simulink model "Pcontrol_perturbed"  (R2024b)
settings: Solver=ode4  StartTime=0.0  StopTime=T  FixedStep=Ts  RelTol=1e-3
values from neighbouring files (symbols this model uses):
  C_perturb = eye(5)    [IP_MACRO.m]
  D_perturb = [0 0 0 0 0]'    [IP_MACRO.m]
  K = lqr(A, B, Qr, Rr)    [IP_MACRO.m]
  x0 = [0.1 1 0.2 0 0]'    [IP_MACRO.m]
undefined symbols (not defined in the file or in its folder): A, B
settings Model: Creator=leita  LastModifiedBy=leita
settings DataIOCC: ReturnWorkspaceOutputs=off

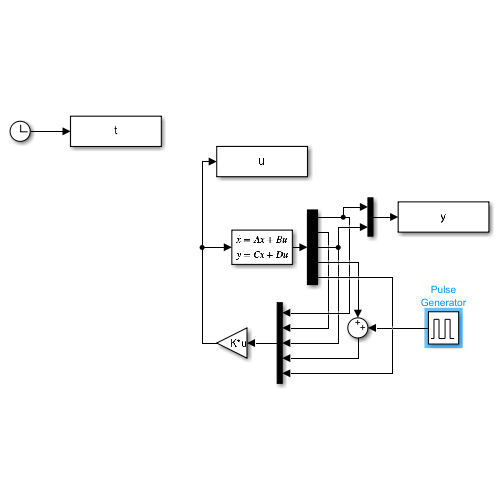
[thumbnail: Simulink's stored preview of the top-level diagram]
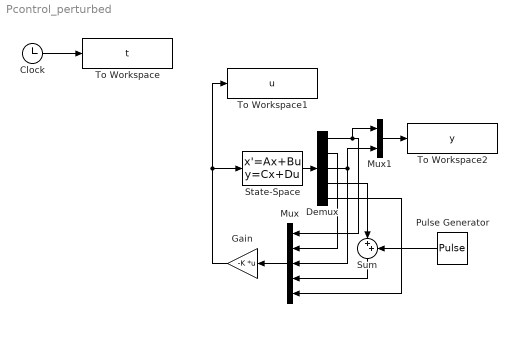
== system Pcontrol_perturbed ==
  Clock : Clock
  Demux : Demux  Outputs=5
  Gain : Gain  Gain=-K  Multiplication=Matrix(K*u)
  Mux : Mux  Inputs=5
  Mux1 : Mux  Inputs=2
  Pulse Generator : DiscretePulseGenerator  PulseType=Time based  Amplitude=5  Period=1  PulseWidth=0.5
  State-Space : StateSpace  A=A  B=B  C=C_perturb  D=D_perturb  InitialCondition=x0
  Sum : Sum  Inputs=|++
  To Workspace : ToWorkspace  VariableName=t  SaveFormat=Timeseries  SampleTime=-1
  To Workspace1 : ToWorkspace  VariableName=u  SaveFormat=Timeseries  SampleTime=-1
  To Workspace2 : ToWorkspace  VariableName=y  SaveFormat=Timeseries  SampleTime=-1
  wires:
  Clock/1 -> To Workspace/1
  Gain/1 -> To Workspace1/1, State-Space/1
  State-Space/1 -> Demux/1
  Pulse Generator/1 -> Sum/2
  Demux/3 -> Mux/3, Mux1/2
  Mux/1 -> Gain/1
  Sum/1 -> Mux/4
  Demux/4 -> Sum/1
  Demux/2 -> Mux/2
  Demux/1 -> Mux1/1, Mux/1
  Mux1/1 -> To Workspace2/1
  Demux/5 -> Mux/5
